simulink model "Lab2spectrum"  (R2016b)
settings: Solver=FixedStepDiscrete  StartTime=0.0  StopTime=0.5  FixedStep=2e-6  RelTol=1e-3  EnableMultiTasking=on
settings Model: Creator=Dennis Silage  LastModifiedBy=Silage
settings DataIOCC: LimitDataPoints=on  SaveFormat=Array  SignalLoggingSaveFormat=ModelDataLogs
settings OptimizationCC: ExpressionDepthLimit=2147483647  InitFltsAndDblsToZero=on  LifeSpan=inf
settings DebuggingCC: UnderspecifiedInitializationDetection=Classic  MergeDetectMultiDrivingBlocksExec=none  FcnCallInpInsideContextMsg=warning  StateNameClashWarn=warning  SFUnexpectedBacktrackingDiag=warning  SFNoUnconditionalDefaultTransitionDiag=warning  SFExecutionAtInitializationDiag=none
settings HardwareCC: ProdBitPerPointer=32  ProdBitPerSizeT=32  ProdBitPerPtrDiffT=32  ProdLargestAtomicFloat=None  ProdIntDivRoundTo=Undefined  ProdEndianess=Unspecified  ProdWordSize=32  ProdHWDeviceType=32-bit Generic
settings ModelReferenceCC: PropagateSignalLabelsOutOfModel=off
settings GRTTargetCC: TargetLangStandard=C89/C90 (ANSI)  GeneratePreprocessorConditionals=Disable all  CombineOutputUpdateFcns=off  GRTInterface=on
settings ConfigComp: CovMetricSettings=dw  CovHtmlReporting=on  CovSaveCumulativeToWorkspaceVar=on  CovSaveSingleToWorkspaceVar=on  CovExternalEMLEnable=off  CovSFcnEnable=off

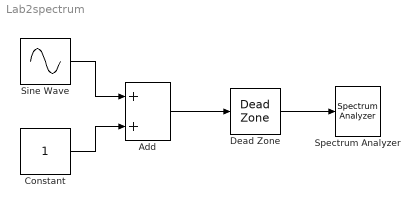
== system Lab2spectrum ==
  Add : Sum
  Constant : Constant
  Dead Zone : DeadZone  LowerValue=-3  UpperValue=3  LinearizeAsGain=off
  Sine Wave : Sin  SineType=Sample based  Amplitude=5  Frequency=2000*pi  Samples=500  SampleTime=2e-6
  Spectrum Analyzer : SpectrumAnalyzer
  wires:
  Dead Zone/1 -> Spectrum Analyzer/1
  Sine Wave/1 -> Add/1
  Constant/1 -> Add/2
  Add/1 -> Dead Zone/1
